simulink model "mls_wzor"  (R2015a)
settings: Solver=ode5  SolverMode=SingleTasking  StartTime=0.0  StopTime=1000  FixedStep=0.001  RelTol=1e-3  AbsTol=1e-6
undefined symbols (not defined in the file): RTDAC4PCIBaseAddress
settings Model: SimulationMode=external  CovSFcnEnable=off  ExtModeEnableFloating=off  ExtModeTrigDuration=40000  ExtModeTrigDirection=either  ExtModeArchiveFileName=exp01.mat  ExtModeArchiveDirName=h:\temp  ExtModeWriteAllDataToWs=on  Creator=Adam Pilat  LastModifiedBy=Student
settings DataIOCC: ExternalInput=[]  InitialState=[]  LimitDataPoints=off  MaxDataPoints=5000  SignalLoggingSaveFormat=ModelDataLogs  SaveOutput=off  SaveTime=off  SignalLoggingName=sigsOut
settings OptimizationCC: BooleanDataType=off  ExpressionDepthLimit=2147483647  InitFltsAndDblsToZero=on
settings DebuggingCC: SaveWithParameterizedLinksMsg=none  UnderspecifiedInitializationDetection=Classic  MergeDetectMultiDrivingBlocksExec=none  SignalResolutionControl=TryResolveAllWithWarning  MultiTaskDSMMsg=warning  MultiTaskCondExecSysMsg=none  IntegerOverflowMsg=none  FcnCallInpInsideContextMsg=UseLocalSettings  StateNameClashWarn=warning  IntegerSaturationMsg=none
settings HardwareCC: ProdBitPerLong=64  ProdBitPerPointer=64  ProdIntDivRoundTo=Zero  ProdEndianess=LittleEndian  ProdWordSize=64  ProdHWDeviceType=Intel->x86-64  TargetBitPerLong=64  TargetBitPerPointer=64  TargetIntDivRoundTo=Zero  TargetEndianess=LittleEndian  TargetWordSize=64  TargetHWDeviceType=Intel->x86-64
settings RTWCC: SystemTargetFile=rtwin.tlc  TemplateMakefile=rtwin.tmf  Description=Real-Time Windows Target
settings RTWinTargetCC: TargetFcnLib=ansi_tfl_tmw.mat  TargetPreCompLibLocation=C:\Program Files\MATLAB\R2015aSP1\toolbox\sldrt\lib\win64  ModelReferenceCompliant=off  CompOptLevelCompliant=off

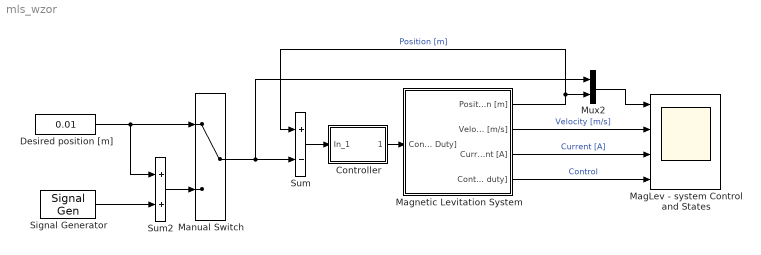
== system mls_wzor ==
  Controller : Subsystem  mask(PID(2) Controller){P=50, I=5, D=2, T0=0.001}
      mask prompts: P "Proportional:"; I "Integral:"; D "Derivative:"; T0 "Sample Time:"
      mask help:
      | Enter Proportional(P), Integral(I), and Derivative(D) and divisor (N) terms.
      | P+I/s+Ds/(1/Ns+1)
      mask Help: This block implements a PID controller where parameters are entered for the Proportional, Integral and Derivative and divisor terms. Unmask this block to see how it works. The derivative term is implemented using an s/(s/N +1)  transfer function block. Making N large can create a "stiff" system.
      mask Display: disp('PID')
  Desired position [m] : Constant  Value=0.01
  MagLev - system Control and States : Scope  NumInputPorts=4
      settings: TimeRange=10.1  YMin=0~-1~0~0  YMax=0.02~1~3~1  SaveName=MLExpData  MaxDataPoints=10000
  Magnetic Levitation System : Subsystem  mask(Magnetic Levitation 1 - System){BA=RTDAC4PCIBaseAddress, T0=0.001}
      mask prompts: BA "Base Address (dec):"; T0 "Sampling period [s]:"
      mask help:
      | MagLev1 - System connection for the real-time operating mode
      | (c) InTeCo 2005
      mask Display: image(imread('MagLev1.tif'))
  Manual Switch : ManualSwitch
  Mux2 : Mux  Inputs=2
  Signal Generator : SignalGenerator  Amplitude=2e-3  Frequency=0.25
  Sum : Sum  Inputs=+-  SaturateOnIntegerOverflow=on  InputSameDT=on  OutDataTypeStr=Inherit: Same as first input
  Sum2 : Sum  SaturateOnIntegerOverflow=on  InputSameDT=on  OutDataTypeStr=Inherit: Same as first input
  wires:
  Magnetic Levitation System/1(Position [m]) -> Mux2/2, Sum/1  "Position [m]"
  Magnetic Levitation System/2(Velocity [m/s]) -> MagLev - system Control and States/2  "Velocity [m/s]"
  Magnetic Levitation System/3(Current [A]) -> MagLev - system Control and States/3  "Current [A]"
  Sum/1 -> Controller/1(In_1)
  Magnetic Levitation System/4(Control [PWM duty]) -> MagLev - system Control and States/4  "Control"
  Desired position [m]/1 -> Sum2/1, Manual Switch/1
  Sum2/1 -> Manual Switch/2
  Signal Generator/1 -> Sum2/2
  Manual Switch/1 -> Sum/2, Mux2/1
  Mux2/1 -> MagLev - system Control and States/1
  Controller/1(Out_1) -> Magnetic Levitation System/1(Control [PWM Duty])

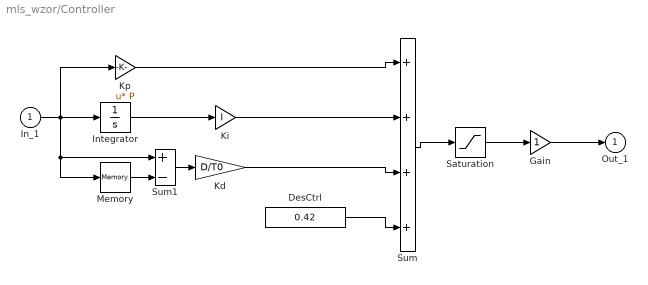
== system mls_wzor/Controller ==
  In_1 : Inport
  DesCtrl : Constant  Value=0.42
  Gain : Gain  SaturateOnIntegerOverflow=on  OutDataTypeStr=Inherit: Same as input  ParamDataTypeStr=Inherit: Same as input
  Integrator : Integrator  InitialCondition=0*4e-5  LimitOutput=on  UpperSaturationLimit=1  LowerSaturationLimit=-1
  Kd : Gain  Gain=D/T0  SaturateOnIntegerOverflow=on  OutDataTypeStr=Inherit: Same as input  ParamDataTypeStr=Inherit: Same as input
  Ki : Gain  Gain=I  SaturateOnIntegerOverflow=on  OutDataTypeStr=Inherit: Same as input  ParamDataTypeStr=Inherit: Same as input
  Kp : Gain  Gain=P  Multiplication=Matrix(u*K)  SaturateOnIntegerOverflow=on  OutDataTypeStr=Inherit: Same as input  ParamDataTypeStr=Inherit: Same as input
  Memory : Memory
  Saturation : Saturate  UpperLimit=1  LowerLimit=0
  Sum : Sum  Inputs=++++  SaturateOnIntegerOverflow=on  InputSameDT=on  OutDataTypeStr=Inherit: Same as first input
  Sum1 : Sum  Inputs=+-  SaturateOnIntegerOverflow=on  InputSameDT=on  OutDataTypeStr=Inherit: Same as first input
  Out_1 : Outport  InitialOutput=0
  wires:
  Ki/1 -> Sum/2
  Integrator/1 -> Ki/1
  Sum/1 -> Saturation/1
  In_1/1 -> Kp/1, Memory/1, Sum1/1, Integrator/1
  Memory/1 -> Sum1/2
  Sum1/1 -> Kd/1
  DesCtrl/1 -> Sum/4
  Saturation/1 -> Gain/1
  Kp/1 -> Sum/1
  Kd/1 -> Sum/3
  Gain/1 -> Out_1/1

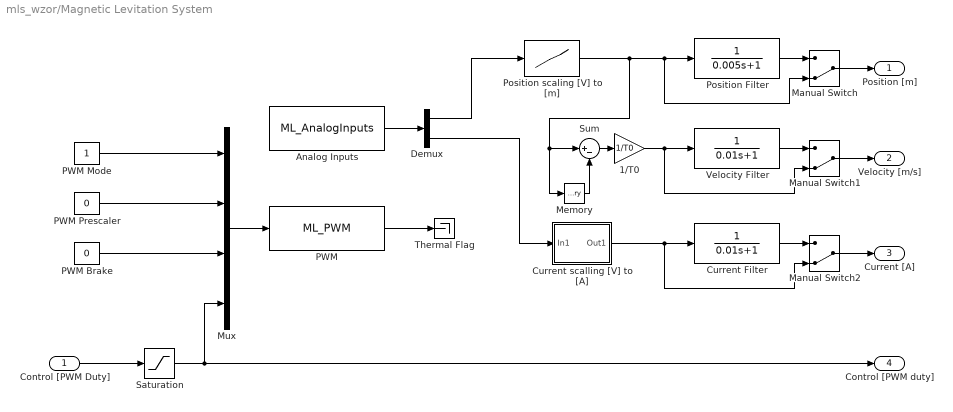
== system mls_wzor/Magnetic Levitation System ==
  Control [PWM Duty] : Inport
  1/T0 : Gain  Gain=1/T0  SaturateOnIntegerOverflow=on  OutDataTypeStr=Inherit: Same as input  ParamDataTypeStr=Inherit: Same as input
  Analog Inputs : S-Function  FunctionName=ML_AnalogInputs  Parameters=BA, [4 2], [1 1], T0
  Current Filter : TransferFcn  Denominator=[0.01 1]
  Current scalling [V] to [A] : Subsystem
      mask Display: plot([0    0.5000    1.0000    1.5000    2.0000    2.5000], [-0.0317    0.4951    1.0302    1.5738    2.1258    2.6863]);
  Demux : Demux  Outputs=2
  Manual Switch : ManualSwitch  CurrentSetting=0
  Manual Switch1 : ManualSwitch  CurrentSetting=0
  Manual Switch2 : ManualSwitch  CurrentSetting=0
  Memory : Memory
  Mux : Mux
  PWM : S-Function  FunctionName=ML_PWM  Parameters=BA, T0
  PWM Brake : Constant  Value=0
  PWM Mode : Constant
  PWM Prescaler : Constant  Value=0
  Position Filter : TransferFcn  Denominator=[0.005 1]
  Position scaling [V] to [m] : Lookup  InputValues=SensorData.Sensor_V(end:-1:1)  Table=SensorData.Distance_m(end:-1:1)  SaturateOnIntegerOverflow=on
  Saturation : Saturate  UpperLimit=1  LowerLimit=0
  Sum : Sum  Inputs=|+-  SaturateOnIntegerOverflow=on  InputSameDT=on  OutDataTypeStr=Inherit: Same as first input
  Thermal Flag : Terminator
  Velocity Filter : TransferFcn  Denominator=[0.01 1]
  Position [m] : Outport
  Velocity [m/s] : Outport  Port=2
  Current [A] : Outport  Port=3
  Control [PWM duty] : Outport  Port=4
  wires:
  Manual Switch1/1 -> Velocity [m/s]/1
  Current Filter/1 -> Manual Switch2/1
  Velocity Filter/1 -> Manual Switch1/1
  Position Filter/1 -> Manual Switch/1
  Demux/1 -> Position scaling [V] to [m]/1
  Demux/2 -> Current scalling [V] to [A]/1(In1)
  Current scalling [V] to [A]/1(Out1) -> Manual Switch2/2, Current Filter/1
  1/T0/1 -> Manual Switch1/2, Velocity Filter/1
  Sum/1 -> 1/T0/1
  Memory/1 -> Sum/2
  Analog Inputs/1 -> Demux/1
  Mux/1 -> PWM/1
  PWM Prescaler/1 -> Mux/2
  PWM Mode/1 -> Mux/1
  PWM/1 -> Thermal Flag/1
  Saturation/1 -> Mux/4, Control [PWM duty]/1
  Control [PWM Duty]/1 -> Saturation/1
  Manual Switch2/1 -> Current [A]/1
  PWM Brake/1 -> Mux/3
  Position scaling [V] to [m]/1 -> Manual Switch/2, Position Filter/1, Memory/1, Sum/1
  Manual Switch/1 -> Position [m]/1

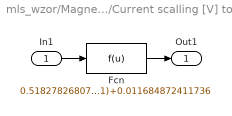
== system mls_wzor/Magnetic Levitation System/Current scalling [V] to [A] ==
  In1 : Inport
  Fcn : Fcn  Expr=0.518278268079857*u(1)+0.011684872411736
  Out1 : Outport
  wires:
  In1/1 -> Fcn/1
  Fcn/1 -> Out1/1
